simulink model "pulse_heating_official_spine_v04"  (R2025b)
settings: Solver=VariableStepAuto  StartTime=0.0  StopTime=0.25  RelTol=1e-3
PreLoadFcn:
  | addpath('C:\Users\ADMIN\Documents\MATLAB\Examples\R2025b\simscapeelectrical\BatteryThermalManagementExample');
  | addpath('C:\Users\ADMIN\Documents\MATLAB\Examples\R2025b\mcb\SIUnitsExample');
  | addpath('C:\Users\ADMIN\Documents\MATLAB\Examples\R2025b\simscapeelectrical\PMSMDriveThermalExample');
  | load_system('PMSMDriveThermal');
  | set_param('PMSMDriveThermal','SimscapeLogType','none','SimscapeLogSimulationStatistics','off');
  | set_param('PMSMDriveThermal','Dirty','off');
InitFcn:
  | % === M4-02A: Clean parameter matching (MO theory PI) ===
  | addpath('C:\Users\ADMIN\Documents\MATLAB\Examples\R2025b\simscapeelectrical\BatteryThermalManagementExample');
  | addpath('C:\Users\ADMIN\Documents\MATLAB\Examples\R2025b\mcb\SIUnitsExample');
  | addpath('C:\Users\ADMIN\Documents\MATLAB\Examples\R2025b\simscapeelectrical\PMSMDriveThermalExample');
  | load_system('PMSMDriveThermal');
  | PMSMDriveThermalData;
  | mcb_pmsm_foc_qep_f28379d_SIUnit_data;
  | clearvars('all');
  | 
  | % --- Construct clean pmsm struct from PMSMDriveThermal ---
  | pmsm = struct();
  | pmsm.Rs = Rs; pmsm.Ld = Ld; pmsm.Lq = Lq; pmsm.p = N; pmsm.FluxPM = PM;
  | pmsm.J = J; pmsm.B = 2.6369e-6; pmsm.I_rated = Imax;
  | pmsm.Ke = PM*N; pmsm.Kt = 1.5*N*PM; pmsm.N_max = 60*fnom/N;
  | pmsm.PositionOffset = 0; pmsm.QEPSlits = 1000;
  | 
  | inverter.V_dc = 70; dataType = 'double';
  | pmsm.N_base = inverter.V_dc / (sqrt(3)*PM*N*2*pi/60);
  | pmsm.T_rated = 1.5*N*PM*Imax;
  | 
  | % --- Timing (PMSMDriveThermal semantics) ---
  | Ts = 2e-6; fsw = 2e3; fc = fsw*10; Tsc = 1/fc;
  | T_pwm = 1/fsw; PWM_frequency = fsw; Ts_simulink = Tsc;
  | Ts_motor = Tsc; Ts_speed = 10*Tsc; Ts_inverter = Tsc;
  | 
  | % --- PI gains via mcb.calcFOCGains (MO theory) ---
  | motor = pmsm; motor.Rs = pmsm.Rs + inverter.R_board;
  | PI_params = mcb.calcFOCGains(motor, Tsc, Ts_speed, SpdLPFltCoeff=0.01);
  | PI_params.delay_Currents = int32(1);
  | PI_params.delay_Position = int32(1);
  | 
  | BatteryThermalManagementInitialization;
  | ambient = 263.15; coolantTemp = 263.15;
  | cellT_ini = ambient*ones(1,Ns*Np); cellT_ini4 = ambient*ones(1,Ns4*Np4);
  | Ns_total = 3*Ns + Ns4; Np_total = Np;
  | R_pack = Ns_total * R0_mat(3,2) / Np_total;
  | I_base_A = AH * Np_total; V_pack_nom = Ns_total * 3.3;
  | 
  | % === M4-01 generalized Reference / Platform contract ===
  | % Values are traceable engineering/platform defaults, not device ratings.
  | ReferenceConfig_ID = 'M4-01-REF-PLATFORM-v02';
  | ReferenceConfig_Source = 'OFFICIAL+ENGINEERING_DEFAULT';
  | ReferenceConfig_Scope = 'generalized_system_integration';
  | HVPath_R = 0.01;
  | DCLink_C = 470e-6;
  | DCLink_V0 = 0;
  | RMS_Window_s = 20/fsw;
  | IGBT_Ron_ref = 1e-3;
  | IGBT_Vf_ref = 1.2;
  | 
  | % Encoder/reference topology provides the static mechanical boundary.
  | OpenLoop_Vabc_Scale = 1;
model workspace (MAT data in the model file):
  control_status_v4d2_partial_duty_code = 6
  diagnostic_frequency_Hz = 50
  drive_status_v4d2_partial_current_code = 6
  kpi_status_v4d2_partial_numeric_code = 6
  kpi_value_unknown = nan
  limit_factor_unknown_code = 99
  limit_margin_unknown_value = nan
  limit_status_v4c_code = 5
  pulse_command_status_code = 6
  pulse_duty_percent = 50
  pulse_id_amplitude_A = 40
  pulse_iq_amplitude_A = 0
  pulse_mode_code = 4
  pulse_phase_delay_s = 0
undefined symbols (not defined in the file or in its folder): DiscIntNeverNeededParam, f_losses, Flowrate_vec, Isc_losses, losses_oc, losses_sc, N, PM, Rs
libraries: fl_lib x38, nesl_utility x35, ee_lib x12, mcbcontrolslib x5, mcbeeMathTransformLib x3, slpidlib x2, mcbhdlpositiondecoderlib x1, eePwmGeneratorTwoLevel x1
(part 1 of 4)
settings Model: Creator=ADMIN  LastModifiedBy=ADMIN
settings DataIOCC: ReturnWorkspaceOutputs=off
settings DebuggingCC: UnderspecifiedInitializationDetection=Classic
settings SimscapeCC: SimscapeLogType=all  SimscapeLogName=simlog_v4e

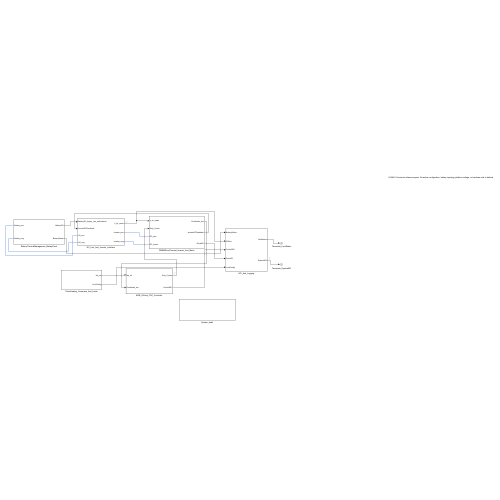
[thumbnail: Simulink's stored preview of the top-level diagram]
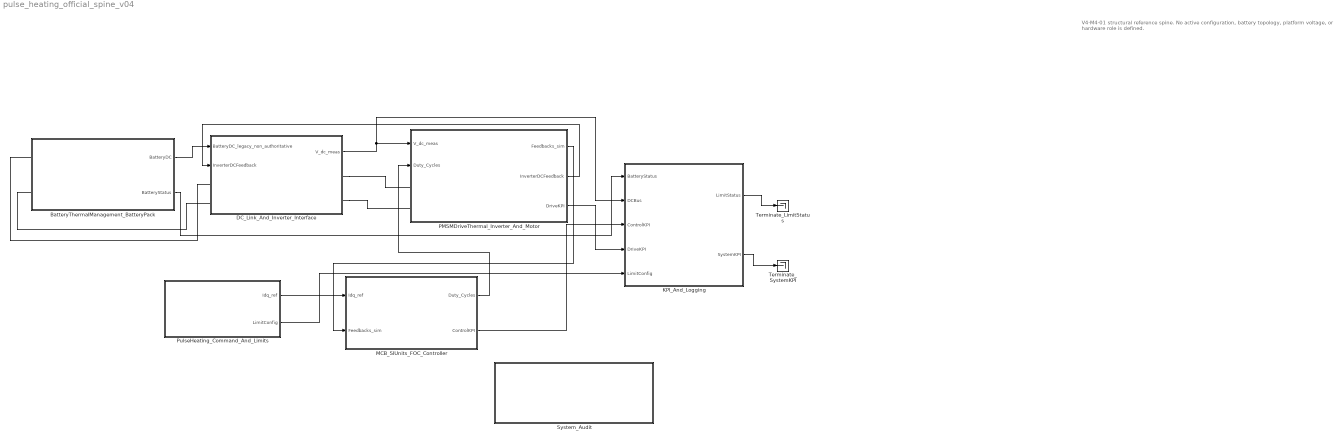
== system pulse_heating_official_spine_v04 ==
  note: V4-M4-01 structural reference spine. No active configuration, battery topology, platform voltage, or hardware role is defined.
  BatteryThermalManagement_BatteryPack : Subsystem
  DC_Link_And_Inverter_Interface : Subsystem
  KPI_And_Logging : Subsystem
  MCB_SIUnits_FOC_Controller : Subsystem
  PMSMDriveThermal_Inverter_And_Motor : Subsystem
  PulseHeating_Command_And_Limits : Subsystem
  System_Audit : Subsystem
  Terminate_LimitStatus : Terminator
  Terminate_SystemKPI : Terminator
  wires:
  BatteryThermalManagement_BatteryPack/1(BatteryDC) -> DC_Link_And_Inverter_Interface/1(BatteryDC_legacy_non_authoritative)
  BatteryThermalManagement_BatteryPack/2(BatteryStatus) -> KPI_And_Logging/1(BatteryStatus)
  PMSMDriveThermal_Inverter_And_Motor/2(InverterDCFeedback) -> DC_Link_And_Inverter_Interface/2(InverterDCFeedback)
  PMSMDriveThermal_Inverter_And_Motor/1(Feedbacks_sim) -> MCB_SIUnits_FOC_Controller/2(Feedbacks_sim)
  PMSMDriveThermal_Inverter_And_Motor/3(DriveKPI) -> KPI_And_Logging/4(DriveKPI)
  PulseHeating_Command_And_Limits/1(Idq_ref) -> MCB_SIUnits_FOC_Controller/1(Idq_ref)
  PulseHeating_Command_And_Limits/2(LimitConfig) -> KPI_And_Logging/5(LimitConfig)
  KPI_And_Logging/1(LimitStatus) -> Terminate_LimitStatus/1
  DC_Link_And_Inverter_Interface/1(V_dc_meas) -> PMSMDriveThermal_Inverter_And_Motor/1(V_dc_meas), KPI_And_Logging/2(DCBus)
  MCB_SIUnits_FOC_Controller/1(Duty_Cycles) -> PMSMDriveThermal_Inverter_And_Motor/2(Duty_Cycles)
  MCB_SIUnits_FOC_Controller/2(ControlKPI) -> KPI_And_Logging/3(ControlKPI)
  KPI_And_Logging/2(SystemKPI) -> Terminate_SystemKPI/1
  connections:
  BatteryThermalManagement_BatteryPack/LConn2 -- DC_Link_And_Inverter_Interface/LConn2
  BatteryThermalManagement_BatteryPack/LConn1 -- DC_Link_And_Inverter_Interface/LConn1
  DC_Link_And_Inverter_Interface/RConn1 -- PMSMDriveThermal_Inverter_And_Motor/LConn1
  DC_Link_And_Inverter_Interface/RConn2 -- PMSMDriveThermal_Inverter_And_Motor/LConn2

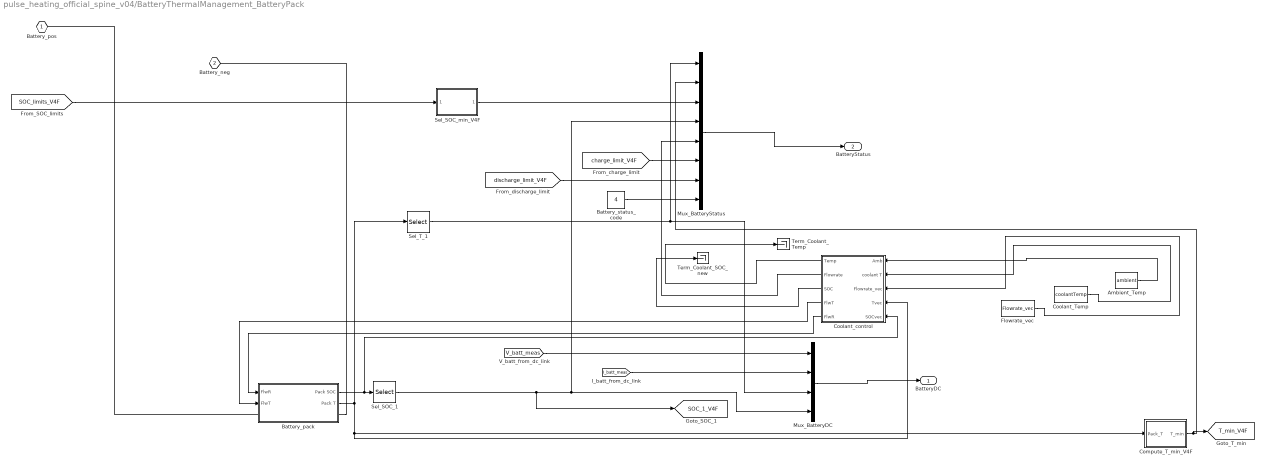
== system pulse_heating_official_spine_v04/BatteryThermalManagement_BatteryPack ==
  Ambient_Temp : Constant  Value=ambient
  Battery_pack : Subsystem
  Battery_status_code : Constant  Value=4
  Compute_T_min_V4F : MATLAB Function  TreatAsAtomicUnit=on
  Coolant_Temp : Constant  Value=coolantTemp
  Coolant_control : Subsystem
  Flowrate_vec : Constant  Value=Flowrate_vec
  Mux_BatteryDC : Mux
  Mux_BatteryStatus : Mux  Inputs=8
  Sel_SOC_1 : Selector  InputPortWidth=42  IndexOptions=Index vector (dialog)  Indices=1  OutputSizes=1
  Sel_SOC_min_V4F : MATLAB Function  TreatAsAtomicUnit=on
  Sel_T_1 : Selector  InputPortWidth=42  IndexOptions=Index vector (dialog)  Indices=1  OutputSizes=1
  Term_Coolant_SOC_new : Terminator
  Term_Coolant_Temp : Terminator
  Battery_pos : PMIOPort  Side=Left
  Battery_neg : PMIOPort  Port=2  Side=Left
  BatteryDC : Outport
  BatteryStatus : Outport  Port=2
  tag scope: SOC_1_V4F=global, T_min_V4F=global
  wires:
  Compute_T_min_V4F/1(T_min) -> [T_min_V4F], Mux_BatteryStatus/2
  Battery_pack/2(Pack T) -> Coolant_control/4(Tvec), Compute_T_min_V4F/1(Pack_T), Sel_T_1/1
  Battery_pack/1(Pack SOC) -> Coolant_control/5(SOCvec), Sel_SOC_1/1
  Flowrate_vec/1 -> Coolant_control/3(Flowrate_vec)
  Coolant_Temp/1 -> Coolant_control/2(coolant T)
  Ambient_Temp/1 -> Coolant_control/1(Amb)
  Coolant_control/1(Temp) -> Term_Coolant_Temp/1
  Coolant_control/3(SOC) -> Term_Coolant_SOC_new/1
  Coolant_control/4(FlwT) -> Battery_pack/2(FlwT)
  Mux_BatteryDC/1 -> BatteryDC/1
  Coolant_control/5(FlwR) -> Battery_pack/1(FlwR)
  Mux_BatteryStatus/1 -> BatteryStatus/1
  Sel_SOC_1/1 -> Mux_BatteryDC/4, Mux_BatteryStatus/4, [SOC_1_V4F]
  [I_batt_meas] -> Mux_BatteryDC/2
  Sel_T_1/1 -> Mux_BatteryStatus/1, Mux_BatteryDC/3
  [V_batt_meas] -> Mux_BatteryDC/1
  Battery_status_code/1 -> Mux_BatteryStatus/8
  [charge_limit_V4F] -> Mux_BatteryStatus/6
  Sel_SOC_min_V4F/1(SOC_min) -> Mux_BatteryStatus/3
  [SOC_limits_V4F] -> Sel_SOC_min_V4F/1(SOC_limits)
  Coolant_control/2(Flowrate) -> Mux_BatteryStatus/5
  [discharge_limit_V4F] -> Mux_BatteryStatus/7
  connections:
  Battery_pack/LConn1 -- Battery_pos/RConn1
  Battery_pack/RConn1 -- Battery_neg/RConn1

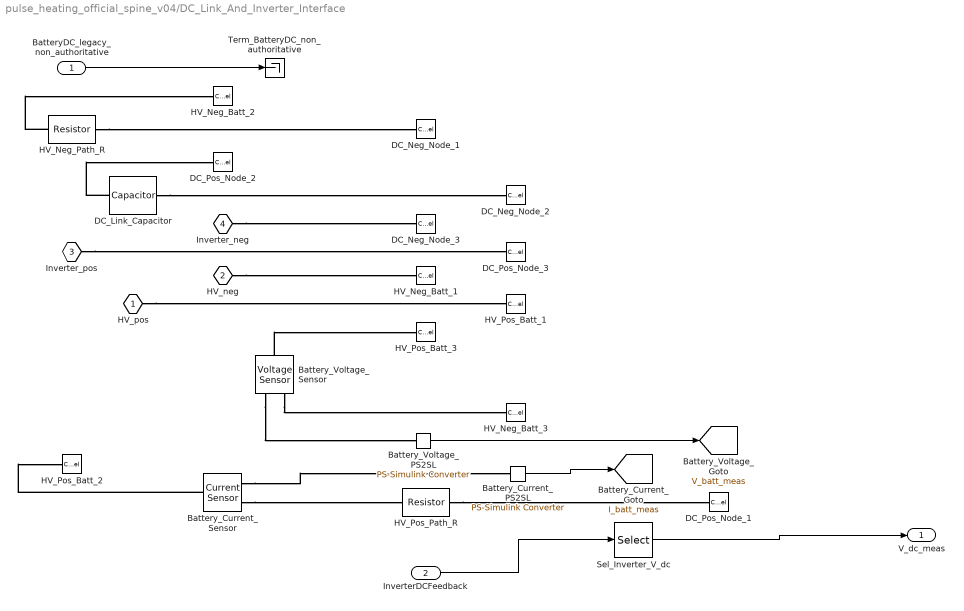
== system pulse_heating_official_spine_v04/DC_Link_And_Inverter_Interface ==
  BatteryDC_legacy_non_authoritative : Inport
  InverterDCFeedback : Inport  Port=2
  Battery_Current_PS2SL : nesl_utility/PS-Simulink Converter  PhysicalDomain=network_engine_domain  SubClassName=ps_output  LeftPortType=input  RightPortType=output  PseudoPeriodic=off  Frequencies=[]  VectorFormat=inherit  Unit=inherit  AffineConversion=off
  Battery_Current_Sensor : fl_lib/Electrical/Electrical Sensors/Current Sensor
  Battery_Voltage_PS2SL : nesl_utility/PS-Simulink Converter  PhysicalDomain=network_engine_domain  SubClassName=ps_output  LeftPortType=input  RightPortType=output  PseudoPeriodic=off  Frequencies=[]  VectorFormat=inherit  Unit=inherit  AffineConversion=off
  Battery_Voltage_Sensor : fl_lib/Electrical/Electrical Sensors/Voltage Sensor
  DC_Link_Capacitor : ee_lib/Passive/Capacitor  cap_option=ee.enum.passive.capacitor.capOption.const  c=DCLink_C F  Cvec=[1e-05, 1e-06] F  Vvec=[0, 10] V  CV_table_symmetry=ee.enum.passive.capacitor.tableSymmetry.yes  f_vec=[1, 10] kHz  DFext_vec=[.8, 1.2]  enable_C_tol=ee.enum.toleranceApplication.none  averaging_period=0 s  C_tol=5  tol_distribution=ee.enum.toleranceDistribution.uniform  nSigma=4  r=0 Ohm  g=0 1/Ohm  enable_operating_limits=ee.enum.enable.no  operating_limit_action=ee.enum.passive.reportOpLim.warn  max_working_voltage_range=[-25, 25] V  power_rating=1 W  maxTemperature=85 degC  thermalEnable=false  thermalMass=1 J/K  i_specify=off  i_priority=None  i=0 A  i_nominal_specify=off  i_nominal_value=1  i_nominal_unit=A  v_specify=off  v_priority=None  v=DCLink_V0 V  v_nominal_specify=off  v_nominal_value=1  v_nominal_unit=V  vc_specify=off  vc_priority=High  vc=DCLink_V0 V  vc_nominal_specify=off  vc_nominal_value=1  vc_nominal_unit=V  T_specify=off  T_priority=None  T=298.15 K  T_nominal_specify=off  T_nominal_value=1  T_nominal_unit=K
  DC_Neg_Node_1 : ConnectionLabel  Label=DC_NEG_NODE
  DC_Neg_Node_2 : ConnectionLabel  Label=DC_NEG_NODE
  DC_Neg_Node_3 : ConnectionLabel  Label=DC_NEG_NODE
  DC_Pos_Node_1 : ConnectionLabel  Label=DC_POS_NODE
  DC_Pos_Node_2 : ConnectionLabel  Label=DC_POS_NODE
  DC_Pos_Node_3 : ConnectionLabel  Label=DC_POS_NODE
  HV_Neg_Batt_1 : ConnectionLabel  Label=HV_NEG_BATT_NODE
  HV_Neg_Batt_2 : ConnectionLabel  Label=HV_NEG_BATT_NODE
  HV_Neg_Batt_3 : ConnectionLabel  Label=HV_NEG_BATT_NODE
  HV_Neg_Path_R : ee_lib/Passive/Resistor  R=HVPath_R Ohm  enable_R_tol=ee.enum.toleranceApplication.none  R_tol=5  tol_distribution=ee.enum.toleranceDistribution.uniform  nSigma=4  enable_operating_limits=ee.enum.enable.no  operating_limit_action=ee.enum.passive.reportOpLim.warn  power_rating=1 W  max_working_voltage=100 V  noise_mode=ee.enum.sources.noise.Disabled  Tdevice=25 degC  sample_time=1e-3 s  repeatability=ee.enum.ic.repeatability.notRepeatable  user_seed=0  auto_seed=3922919431  power_derating_T1=70 degC  power_derating_T2=155 degC  operating_temperature_range_vec=[-50, 150] degC  alpha=3.93e-3 1/K  Tmeas=25 degC  thermal_mass=100 J/K  temperature_specify=off  temperature_priority=High  temperature=298.15 K  temperature_nominal_specify=off  temperature_nominal_value=1  temperature_nominal_unit=K
  HV_Pos_Batt_1 : ConnectionLabel  Label=HV_POS_BATT_NODE
  HV_Pos_Batt_2 : ConnectionLabel  Label=HV_POS_BATT_NODE
  HV_Pos_Batt_3 : ConnectionLabel  Label=HV_POS_BATT_NODE
  HV_Pos_Path_R : ee_lib/Passive/Resistor  R=HVPath_R Ohm  enable_R_tol=ee.enum.toleranceApplication.none  R_tol=5  tol_distribution=ee.enum.toleranceDistribution.uniform  nSigma=4  enable_operating_limits=ee.enum.enable.no  operating_limit_action=ee.enum.passive.reportOpLim.warn  power_rating=1 W  max_working_voltage=100 V  noise_mode=ee.enum.sources.noise.Disabled  Tdevice=25 degC  sample_time=1e-3 s  repeatability=ee.enum.ic.repeatability.notRepeatable  user_seed=0  auto_seed=545404223  power_derating_T1=70 degC  power_derating_T2=155 degC  operating_temperature_range_vec=[-50, 150] degC  alpha=3.93e-3 1/K  Tmeas=25 degC  thermal_mass=100 J/K  temperature_specify=off  temperature_priority=High  temperature=298.15 K  temperature_nominal_specify=off  temperature_nominal_value=1  temperature_nominal_unit=K
  Sel_Inverter_V_dc : Selector  InputPortWidth=4  IndexOptions=Index vector (dialog)  Indices=1  OutputSizes=1
  Term_BatteryDC_non_authoritative : Terminator
  HV_pos : PMIOPort  Side=Left
  HV_neg : PMIOPort  Port=2  Side=Left
  Inverter_pos : PMIOPort  Port=3  Side=Right
  Inverter_neg : PMIOPort  Port=4  Side=Right
  V_dc_meas : Outport
  tag scope: I_batt_meas=global, V_batt_meas=global
  wires:
  BatteryDC_legacy_non_authoritative/1 -> Term_BatteryDC_non_authoritative/1
  InverterDCFeedback/1 -> Sel_Inverter_V_dc/1
  Sel_Inverter_V_dc/1 -> V_dc_meas/1
  Battery_Current_PS2SL/1 -> [I_batt_meas]
  Battery_Voltage_PS2SL/1 -> [V_batt_meas]
  connections:
  Battery_Current_Sensor/RConn2 -- HV_Pos_Path_R/LConn1
  Battery_Current_Sensor/RConn1 -- Battery_Current_PS2SL/LConn1
  Battery_Voltage_Sensor/RConn1 -- Battery_Voltage_PS2SL/LConn1
  HV_pos/RConn1 -- HV_Pos_Batt_1/LConn1
  Battery_Current_Sensor/LConn1 -- HV_Pos_Batt_2/LConn1
  Battery_Voltage_Sensor/LConn1 -- HV_Pos_Batt_3/LConn1
  HV_neg/RConn1 -- HV_Neg_Batt_1/LConn1
  HV_Neg_Path_R/LConn1 -- HV_Neg_Batt_2/LConn1
  Battery_Voltage_Sensor/RConn2 -- HV_Neg_Batt_3/LConn1
  HV_Pos_Path_R/RConn1 -- DC_Pos_Node_1/LConn1
  DC_Link_Capacitor/LConn1 -- DC_Pos_Node_2/LConn1
  Inverter_pos/RConn1 -- DC_Pos_Node_3/LConn1
  HV_Neg_Path_R/RConn1 -- DC_Neg_Node_1/LConn1
  DC_Link_Capacitor/RConn1 -- DC_Neg_Node_2/LConn1
  Inverter_neg/RConn1 -- DC_Neg_Node_3/LConn1

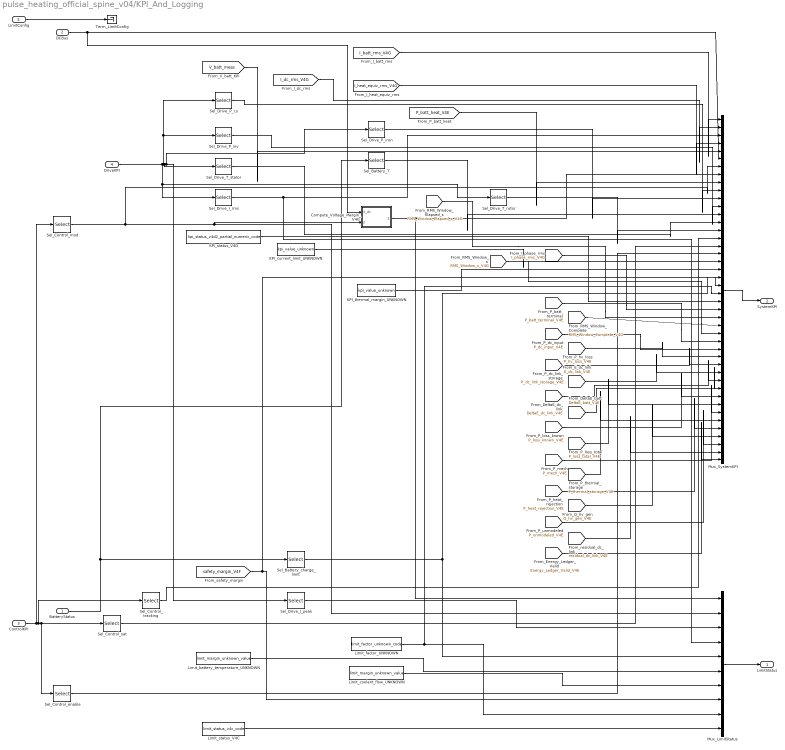
== system pulse_heating_official_spine_v04/KPI_And_Logging ==
  BatteryStatus : Inport
  DCBus : Inport  Port=2
  ControlKPI : Inport  Port=3
  DriveKPI : Inport  Port=4
  LimitConfig : Inport  Port=5
  Compute_Voltage_Margin_V4G : MATLAB Function  TreatAsAtomicUnit=on
  KPI_current_limit_UNKNOWN : Constant  Value=kpi_value_unknown
  KPI_status_V4D : Constant  Value=kpi_status_v4d2_partial_numeric_code
  KPI_thermal_margin_UNKNOWN : Constant  Value=kpi_value_unknown
  Limit_battery_temperature_UNKNOWN : Constant  Value=limit_margin_unknown_value
  Limit_coolant_flow_UNKNOWN : Constant  Value=limit_margin_unknown_value
  Limit_factor_UNKNOWN : Constant  Value=limit_factor_unknown_code
  Limit_status_V4C : Constant  Value=limit_status_v4c_code
  Mux_LimitStatus : Mux  Inputs=10
  Mux_SystemKPI : Mux  Inputs=44
  Sel_Battery_T : Selector  InputPortWidth=8  IndexOptions=Index vector (dialog)  Indices=1  OutputSizes=1
  Sel_Battery_charge_limit : Selector  InputPortWidth=8  IndexOptions=Index vector (dialog)  Indices=6  OutputSizes=1
  Sel_Control_enable : Selector  InputPortWidth=5  IndexOptions=Index vector (dialog)  Indices=4  OutputSizes=1
  Sel_Control_mod : Selector  InputPortWidth=5  IndexOptions=Index vector (dialog)  Indices=2  OutputSizes=1
  Sel_Control_sat : Selector  InputPortWidth=5  IndexOptions=Index vector (dialog)  Indices=3  OutputSizes=1
  Sel_Control_tracking : Selector  InputPortWidth=5  IndexOptions=Index vector (dialog)  Indices=1  OutputSizes=1
  Sel_Drive_I_peak : Selector  InputPortWidth=8  IndexOptions=Index vector (dialog)  Indices=2  OutputSizes=1
  Sel_Drive_I_rms : Selector  InputPortWidth=8  IndexOptions=Index vector (dialog)  Indices=1  OutputSizes=1
  Sel_Drive_P_cu : Selector  InputPortWidth=8  IndexOptions=Index vector (dialog)  Indices=3  OutputSizes=1
  Sel_Drive_P_inv : Selector  InputPortWidth=8  IndexOptions=Index vector (dialog)  Indices=5  OutputSizes=1
  Sel_Drive_P_iron : Selector  InputPortWidth=8  IndexOptions=Index vector (dialog)  Indices=4  OutputSizes=1
  Sel_Drive_T_rotor : Selector  InputPortWidth=8  IndexOptions=Index vector (dialog)  Indices=7  OutputSizes=1
  Sel_Drive_T_stator : Selector  InputPortWidth=8  IndexOptions=Index vector (dialog)  Indices=6  OutputSizes=1
  Term_LimitConfig : Terminator
  LimitStatus : Outport
  SystemKPI : Outport  Port=2
  wires:
  Sel_Drive_P_cu/1 -> Mux_SystemKPI/10
  BatteryStatus/1 -> Sel_Battery_T/1, Sel_Battery_charge_limit/1
  LimitConfig/1 -> Term_LimitConfig/1
  Sel_Control_sat/1 -> Mux_SystemKPI/17
  ControlKPI/1 -> Sel_Control_enable/1, Sel_Control_sat/1, Sel_Control_tracking/1, Sel_Control_mod/1
  DCBus/1 -> Mux_SystemKPI/6, Compute_Voltage_Margin_V4G/1(V_dc)
  DriveKPI/1 -> Sel_Drive_T_rotor/1, Sel_Drive_I_rms/1, Sel_Drive_I_peak/1, Sel_Drive_P_iron/1, Sel_Drive_T_stator/1, Sel_Drive_P_inv/1, Sel_Drive_P_cu/1
  Sel_Control_mod/1 -> Compute_Voltage_Margin_V4G/2(mod_index), Mux_LimitStatus/2, Mux_SystemKPI/7
  Limit_status_V4C/1 -> Mux_LimitStatus/10
  Sel_Control_tracking/1 -> Mux_SystemKPI/16
  Sel_Control_enable/1 -> Mux_SystemKPI/18
  [I_batt_rms_V4G] -> Mux_SystemKPI/1
  [I_dc_rms_V4G] -> Mux_SystemKPI/2
  [I_heat_equiv_rms_V4G] -> Mux_SystemKPI/4
  [V_batt_meas] -> Mux_SystemKPI/5
  Mux_SystemKPI/1 -> SystemKPI/1
  [P_batt_heat_V4E] -> Mux_SystemKPI/9
  Sel_Drive_P_iron/1 -> Mux_SystemKPI/11
  Sel_Drive_P_inv/1 -> Mux_SystemKPI/12
  Sel_Battery_T/1 -> Mux_SystemKPI/13
  Sel_Drive_T_stator/1 -> Mux_SystemKPI/14
  Sel_Drive_T_rotor/1 -> Mux_SystemKPI/15
  KPI_status_V4D/1 -> Mux_SystemKPI/24
  Sel_Drive_I_rms/1 -> Mux_SystemKPI/3, Mux_LimitStatus/4
  Compute_Voltage_Margin_V4G/1(V_margin) -> Mux_LimitStatus/1, Mux_SystemKPI/8
  KPI_current_limit_UNKNOWN/1 -> Mux_SystemKPI/19
  KPI_thermal_margin_UNKNOWN/1 -> Mux_SystemKPI/20
  Limit_coolant_flow_UNKNOWN/1 -> Mux_LimitStatus/7
  Sel_Battery_charge_limit/1 -> Mux_LimitStatus/5, Mux_SystemKPI/21
  Mux_LimitStatus/1 -> LimitStatus/1
  [safety_margin_V4F] -> Mux_LimitStatus/8, Mux_SystemKPI/22
  Sel_Drive_I_peak/1 -> Mux_LimitStatus/3
  Limit_factor_UNKNOWN/1 -> Mux_SystemKPI/23, Mux_LimitStatus/9
  Limit_battery_temperature_UNKNOWN/1 -> Mux_LimitStatus/6
  [I_phase_rms_V4G] -> Mux_SystemKPI/25
  [RMS_Window_Elapsed_s_V4G] -> Mux_SystemKPI/26
  [RMS_Window_Complete_V4G] -> Mux_SystemKPI/27
  [RMS_Window_s_V4G] -> Mux_SystemKPI/28
  [P_batt_terminal_V4E] -> Mux_SystemKPI/29
  [P_dc_input_V4E] -> Mux_SystemKPI/30
  [P_hv_loss_V4E] -> Mux_SystemKPI/31
  [P_dc_link_storage_V4E] -> Mux_SystemKPI/32
  [E_dc_link_V4E] -> Mux_SystemKPI/33
  [DeltaE_dc_link_V4E] -> Mux_SystemKPI/34
  [DeltaE_batt_V4E] -> Mux_SystemKPI/35
  [P_loss_known_V4E] -> Mux_SystemKPI/36
  [P_loss_total_V4E] -> Mux_SystemKPI/37
  [P_mech_V4E] -> Mux_SystemKPI/38
  [P_thermal_storage_V4E] -> Mux_SystemKPI/39
  [P_heat_rejection_V4E] -> Mux_SystemKPI/40
  [Q_hv_gen_V4E] -> Mux_SystemKPI/41
  [P_unmodeled_V4E] -> Mux_SystemKPI/42
  [residual_dc_link_V4E] -> Mux_SystemKPI/43
  [Energy_Ledger_Valid_V4E] -> Mux_SystemKPI/44

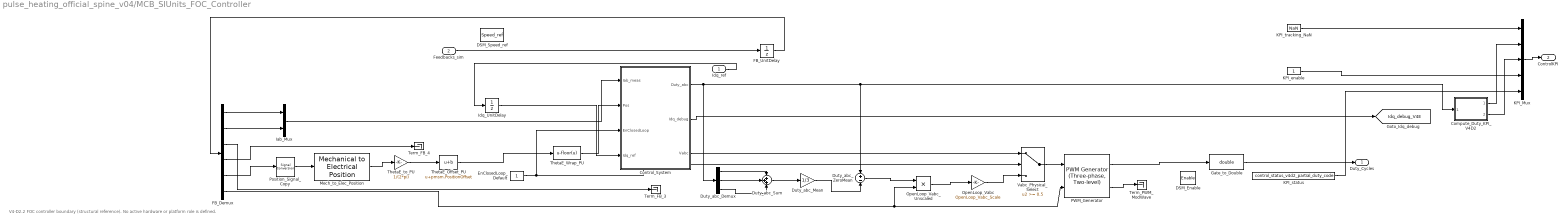
== system pulse_heating_official_spine_v04/MCB_SIUnits_FOC_Controller ==
  note: V4-D2.2 FOC controller boundary (structural reference). No active hardware or platform role is defined.
  Idq_ref : Inport
  Feedbacks_sim : Inport  Port=2
  Compute_Duty_KPI_V4D2 : MATLAB Function  TreatAsAtomicUnit=on
  Control_System : Subsystem  TreatAsAtomicUnit=on
  DSM_Enable : DataStoreMemory  DataStoreName=Enable  WriteAfterWriteMsg=warning  InitialValue=1  ShowAdditionalParam=off
  DSM_Speed_ref : DataStoreMemory  DataStoreName=Speed_ref  WriteAfterWriteMsg=warning  ShowAdditionalParam=off
  Duty_abc_Demux : Demux  Outputs=3
  Duty_abc_Mean : Gain  Gain=1/3
  Duty_abc_Sum : Sum  Inputs=+++
  Duty_abc_ZeroMean : Sum  Inputs=+-
  EnClosedLoop_Default : Constant
  FB_Demux : Demux  Outputs=6
  FB_UnitDelay : UnitDelay  InitialCondition=[0;0;0;0;0;inverter.V_dc]  SampleTime=Tsc  HasFrameUpgradeWarning=on
  Gate_to_Double : DataTypeConversion  OutDataTypeStr=double
  Iab_Mux : Mux  Inputs=2
  Idq_UnitDelay : UnitDelay  SampleTime=Tsc  HasFrameUpgradeWarning=on
  KPI_Mux : Mux  Inputs=5
  KPI_enable : Constant
  KPI_status : Constant  Value=control_status_v4d2_partial_duty_code
  KPI_tracking_NaN : Constant  Value=NaN
  Mech_to_Elec_Position : mcbhdlpositiondecoderlib/Mechanical to Electrical Position  PolePairsInputType=Specify via dialog  NrPP=pmsm.p  selectedRange=Radians  MechOfstInputType=Specify via dialog  mechOffsetIn=0  maxAngleIn=2*pi  InputDataType=double  VariantSelect=floating-point
      settings: LibrarySourceBlock=mcbhdllib/Sensor Decoders/Mechanical to Electrical Position
  OpenLoop_Vabc : Gain  Gain=OpenLoop_Vabc_Scale
  OpenLoop_Vabc_Unscaled : Product  Inputs=**
  PWM_Generator : eePwmGeneratorTwoLevel/PWM Generator (Three-phase, Two-level)  PWMMode=Continuous PWM (CPWM)  CPWMMode=SVM: space vector modulation  DPWMMode=60 DPWM: 60 degree discontinuous PWM  fsw=fsw  Ts=Ts
  Position_Signal_Copy : SignalConversion  OverrideOpt=off
  Term_FB_3 : Terminator
  Term_FB_4 : Terminator
  Term_PWM_ModWave : Terminator
  ThetaE_Offset_PU : Bias  Bias=pmsm.PositionOffset
  ThetaE_Wrap_PU : Fcn  Expr=u-floor(u)
  ThetaE_to_PU : Gain  Gain=1/(2*pi)
  Vabc_Physical_Select : Switch  Threshold=0.5
  Duty_Cycles : Outport
  ControlKPI : Outport  Port=2
  tag scope: Idq_debug_V4E=global
  wires:
  Position_Signal_Copy/1 -> Mech_to_Elec_Position/1
  FB_Demux/5 -> Position_Signal_Copy/1
  Gate_to_Double/1 -> Duty_Cycles/1
  PWM_Generator/1 -> Gate_to_Double/1
  PWM_Generator/2 -> Term_PWM_ModWave/1
  Control_System/3(Vabc) -> Vabc_Physical_Select/1
  KPI_status/1 -> KPI_Mux/5
  KPI_enable/1 -> KPI_Mux/4
  Compute_Duty_KPI_V4D2/2(sat_flag) -> KPI_Mux/3
  Compute_Duty_KPI_V4D2/1(mod_index) -> KPI_Mux/2
  KPI_Mux/1 -> ControlKPI/1
  Control_System/2(Idq_debug) -> [Idq_debug_V4E]
  Idq_UnitDelay/1 -> Control_System/4(Idq_ref)
  EnClosedLoop_Default/1 -> Control_System/3(EnClosedLoop), Vabc_Physical_Select/2
  Iab_Mux/1 -> Control_System/1(Iab_meas)
  Idq_ref/1 -> Idq_UnitDelay/1
  KPI_tracking_NaN/1 -> KPI_Mux/1
  FB_Demux/6 -> PWM_Generator/2, OpenLoop_Vabc_Unscaled/2
  FB_Demux/4 -> Term_FB_4/1
  Control_System/1(Duty_abc) -> Compute_Duty_KPI_V4D2/1(duty_abc), Duty_abc_ZeroMean/1, Duty_abc_Demux/1
  FB_Demux/3 -> Term_FB_3/1
  FB_Demux/2 -> Iab_Mux/2
  FB_UnitDelay/1 -> FB_Demux/1
  FB_Demux/1 -> Iab_Mux/1
  Feedbacks_sim/1 -> FB_UnitDelay/1
  Mech_to_Elec_Position/1 -> ThetaE_to_PU/1
  ThetaE_to_PU/1 -> ThetaE_Offset_PU/1
  ThetaE_Offset_PU/1 -> ThetaE_Wrap_PU/1
  ThetaE_Wrap_PU/1 -> Control_System/2(Pos)
  Duty_abc_Demux/1 -> Duty_abc_Sum/1
  Duty_abc_Demux/2 -> Duty_abc_Sum/2
  Duty_abc_Demux/3 -> Duty_abc_Sum/3
  Duty_abc_Sum/1 -> Duty_abc_Mean/1
  Duty_abc_Mean/1 -> Duty_abc_ZeroMean/2
  Duty_abc_ZeroMean/1 -> OpenLoop_Vabc_Unscaled/1
  OpenLoop_Vabc_Unscaled/1 -> OpenLoop_Vabc/1
  OpenLoop_Vabc/1 -> Vabc_Physical_Select/3
  Vabc_Physical_Select/1 -> PWM_Generator/1

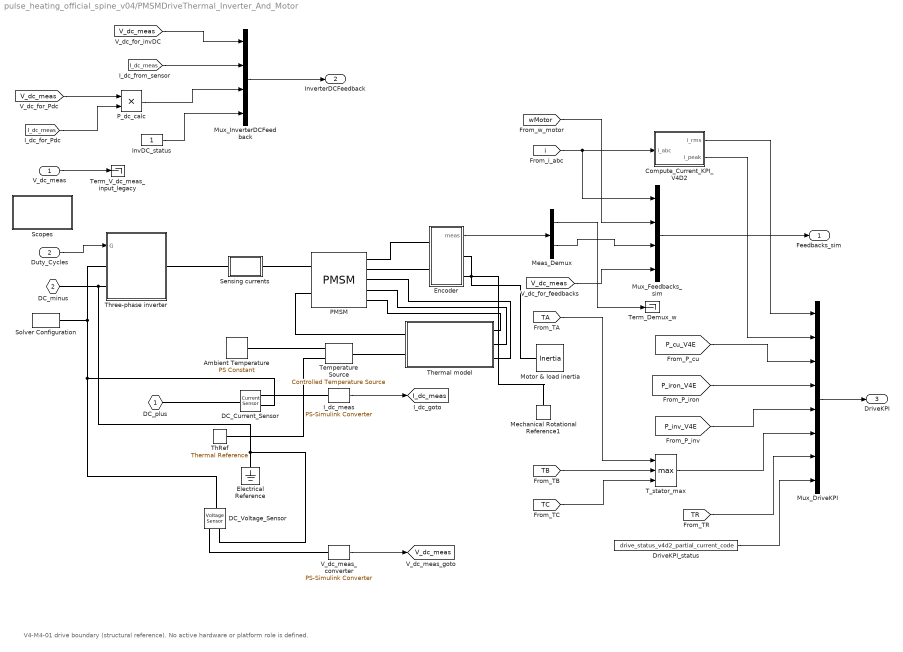
== system pulse_heating_official_spine_v04/PMSMDriveThermal_Inverter_And_Motor ==
  note: V4-M4-01 drive boundary (structural reference). No active hardware or platform role is defined.
  V_dc_meas : Inport
  Duty_Cycles : Inport  Port=2
  Ambient Temperature : fl_lib/Physical Signals/Sources/PS Constant  constant=300.15 K
  Compute_Current_KPI_V4D2 : MATLAB Function  TreatAsAtomicUnit=on
  DC_Current_Sensor : fl_lib/Electrical/Electrical Sensors/Current Sensor
  DC_Voltage_Sensor : fl_lib/Electrical/Electrical Sensors/Voltage Sensor
  DriveKPI_status : Constant  Value=drive_status_v4d2_partial_current_code
  Electrical Reference : fl_lib/Electrical/Electrical Elements/Electrical Reference
  Encoder : Subsystem
  I_dc_meas : nesl_utility/PS-Simulink Converter  PhysicalDomain=network_engine_domain  SubClassName=ps_output  LeftPortType=input  RightPortType=output  PseudoPeriodic=off  Frequencies=[]  VectorFormat=inherit  Unit=inherit  AffineConversion=off
  InvDC_status : Constant
  Meas_Demux : Demux  Outputs=2
  Mechanical Rotational Reference1 : fl_lib/Mechanical/Rotational Elements/Mechanical Rotational Reference
  Motor & load inertia : fl_lib/Mechanical/Rotational Elements/Inertia  inertia=J kg*m^2  num_ports=foundation.enum.numPorts2.one  w_specify=on  w_priority=High  w=0 rpm  w_nominal_specify=off  w_nominal_value=1  w_nominal_unit=rad/s  t_specify=off  t_priority=High  t=0 N*m  t_nominal_specify=off  t_nominal_value=1  t_nominal_unit=N*m
  Mux_DriveKPI : Mux  Inputs=8
  Mux_Feedbacks_sim : Mux
  Mux_InverterDCFeedback : Mux
  PMSM : ee_lib/Electromechanical/Permanent Magnet/PMSM  port_option=ee.enum.threePhasePort.composite  winding_type=ee.enum.statorconnection.wye  machine_param=ee.enum.pmsm.parameterization.constant  nPolePairs=N  pmflux_param=ee.enum.pmflux.fluxlinkage  pm_flux_linkage=PM Wb  torque_constant=0.18 N*m/A  back_emf_constant=0.18 V/(rad/s)  stator_param=ee.enum.statorparam.LdLqL0  Ld=Ld H  Lq=Lq H  idVec=[-200, 0, 200] A  iqVec=[-200, 0, 200] A  LdMatrix=0.0002 * ones(3, 3) H  LqMatrix=0.0002 * ones(3, 3) H  PmMatrix=0.1 * ones(3, 3) Wb  ktMatrix=0.18 * ones(3, 3) N*m/A  keMatrix=0.18 * ones(3, 3) V/(rad/s)  L0=L0 H  Ls=0.0002 H  Lm=0.00002 H  Ms=0.00002 H  Rs=Rs Ohm  zero_sequence=ee.enum.park.zerosequence.exclude  axes_param=ee.enum.rotorangle.qaxis  loss_param=ee.enum.ironloss.empirical  losses_oc=losses_oc W  losses_sc=losses_sc W  f_losses=f_losses Hz  Isc_losses=Isc_losses A  J=0 kg*m^2  lam=0 N*m/(rad/s)  i_d_specify=off  i_d_priority=None  i_d=0 A  i_d_nominal_specify=off  i_d_nominal_value=1  i_d_nominal_unit=A  i_q_specify=off  i_q_priority=None  i_q=0 A  i_q_nominal_specify=off  i_q_nominal_value=1  i_q_nominal_unit=A  torque_specify=off  torque_priority=None  torque=0 N*m  torque_nominal_specify=off  torque_nominal_value=1  torque_nominal_unit=N*m  angular_velocity_specify=on  angular_velocity_priority=None  angular_velocity=0 rpm  angular_velocity_nominal_specify=off  angular_velocity_nominal_value=1  angular_velocity_nominal_unit=rpm  angular_position_specify=on  angular_position_priority=High  angular_position=0 rad  angular_position_nominal_specify=off  angular_position_nominal_value=1  angular_position_nominal_unit=deg  alpha=alpha 1/K  alpha_flux=alpha_flux 1/K  Tmeas=Tmeas K  stator_thermal_mass=stator_thermal_mass J/K  rotor_thermal_mass=rotor_thermal_mass J/K  Rm_percent_rotor=Rm_percent_rotor  Rd_percent_rotor=Rd_percent_rotor  temperatureA_specify=off  temperatureA_priority=High  temperatureA=25 degC  temperatureA_nominal_specify=off  temperatureA_nominal_value=1  temperatureA_nominal_unit=degC  temperatureB_specify=off  temperatureB_priority=High  temperatureB=25 degC  temperatureB_nominal_specify=off  temperatureB_nominal_value=1  temperatureB_nominal_unit=degC  temperatureC_specify=off  temperatureC_priority=High  temperatureC=25 degC  temperatureC_nominal_specify=off  temperatureC_nominal_value=1  temperatureC_nominal_unit=degC  temperatureR_specify=off  temperatureR_priority=High  temperatureR=25 degC  temperatureR_nominal_specify=off  temperatureR_nominal_value=1  temperatureR_nominal_unit=degC
      settings: InternalSimscapePortConfiguration="{\"Bottom\":[],\"Left\":[{\"id\":\"N\",\"label\":\"~\",\"type\":\"foundation.electrical.three_phase\"},{\"id\":\"HR\",\"label\":\"HR\",\"type\":\"foundation.thermal.thermal\"}],\"Right\":[{\"id\":\"R\",\"label\":\"R\",\"type\":\"foundation.mechanical.rotational.rotational\"},{\"id\":\"C\",\"label\":\"C\",\"type\":\"foundation.mechanical.rotational.rotational\"},{\"id\":\"HA\",\"label\":\"HA\",\"type\":\"foundation.thermal.thermal\"},{\"id\":\"HB\",\"label\":\"HB\",\"type\":\"foundation.thermal.thermal\"},{\"id\":\"HC\",\"label\":\"HC\",\"type\":\"foundation.thermal.thermal\"}],\"Top\":[]}"
  P_dc_calc : Product
  Scopes : Subsystem
  Sensing currents : Subsystem
      mask Display: disp('i')
  Solver Configuration : nesl_utility/Solver Configuration  PhysicalDomain=network_engine_domain  SubClassName=solver  LeftPortType=input  RightPortType=generic  Tones=[]  Harmonics=[]  SimulateNoise=off  Profile=off  UseLocalSampling=off  EnableSwitchedLinearOptims=on  FrequencyDomain=off  UseCCode=off  RelTol=0.001  AbsTol=1e-06  MinStep=1e-09  ToWorkspace=off  RevertToSquareIcSolve=off  NumHomotopyIterations=100  PhasorMode=off  PhasorModeNumHarmonics=1  ConsistencySolver=NEWTON_FTOL  IndexReductionMethod=DerivativeReplacement  DoDC=off  ResidualTolerance=1e-9  ConsistencyTolSource=GLOBAL  ConsistencyAbsTol=0.001  ConsistencyRelTol=0.001  ConsistencyTolFactor=0.001  UseLocalSolver=on  LocalSolverChoice=NE_BACKWARD_EULER_ADVANCER  ResolveIndetEquations=on  FunctionEvalNumThread=1  LocalSolverSampleTime=Ts  DoFixedCost=on  MaxNonlinIter=6  MaxModeIter=2  ComputeImpulses=off  ImpulseIterations=2  LinearAlgebra=auto  LinearAlgebraNumThread=0  EquationFormulation=NE_TIME_EF  DelaysMemoryBudget=1024  AutomaticFiltering=on  FilteringTimeConstant=0.001  PartitionStorageMethod=AS_NEEDED  PartitionMemoryBudget=1024  PartitionMethod=FAST  MultibodyUseLocalSolver=off  MultibodyLocalSolverChoice=ODE1  MultibodyLocalSolverSampleTime=0.001
  T_stator_max : MinMax  Function=max  Inputs=3
  Temperature Source : fl_lib/Thermal/Thermal Sources/Controlled Temperature Source
  Term_Demux_w : Terminator
  Term_V_dc_meas_input_legacy : Terminator
  ThRef : fl_lib/Thermal/Thermal Elements/Thermal Reference
  Thermal model : Subsystem  Tag=PublishSubsystem
  Three-phase inverter : Subsystem
  V_dc_meas_converter : nesl_utility/PS-Simulink Converter  PhysicalDomain=network_engine_domain  SubClassName=ps_output  LeftPortType=input  RightPortType=output  PseudoPeriodic=off  Frequencies=[]  VectorFormat=inherit  Unit=inherit  AffineConversion=off
  DC_plus : PMIOPort  Side=Left
  DC_minus : PMIOPort  Port=2  Side=Left
  Feedbacks_sim : Outport
  InverterDCFeedback : Outport  Port=2
  DriveKPI : Outport  Port=3
  tag scope: I_dc_meas=global, V_dc_meas=global
  wires:
  [V_dc_meas] -> Mux_InverterDCFeedback/1
  [V_dc_meas] -> P_dc_calc/1
  [I_dc_meas] -> P_dc_calc/2
  [I_dc_meas] -> Mux_InverterDCFeedback/2
  V_dc_meas/1 -> Term_V_dc_meas_input_legacy/1
  Duty_Cycles/1 -> Three-phase inverter/1(G)
  P_dc_calc/1 -> Mux_InverterDCFeedback/3
  InvDC_status/1 -> Mux_InverterDCFeedback/4
  V_dc_meas_converter/1 -> [V_dc_meas]
  [P_iron_V4E] -> Mux_DriveKPI/4
  T_stator_max/1 -> Mux_DriveKPI/6
  Mux_InverterDCFeedback/1 -> InverterDCFeedback/1
  DriveKPI_status/1 -> Mux_DriveKPI/8
  Meas_Demux/2 -> Mux_Feedbacks_sim/3
  Meas_Demux/1 -> Term_Demux_w/1
  [TA] -> T_stator_max/1
  [TB] -> T_stator_max/2
  I_dc_meas/1 -> [I_dc_meas]
  Encoder/1(meas) -> Meas_Demux/1
  [wMotor] -> Mux_Feedbacks_sim/2
  [i] -> Mux_Feedbacks_sim/1, Compute_Current_KPI_V4D2/1(i_abc)
  [V_dc_meas] -> Mux_Feedbacks_sim/4
  [TC] -> T_stator_max/3
  Compute_Current_KPI_V4D2/1(i_rms) -> Mux_DriveKPI/1
  Compute_Current_KPI_V4D2/2(i_peak) -> Mux_DriveKPI/2
  Mux_Feedbacks_sim/1 -> Feedbacks_sim/1
  [P_cu_V4E] -> Mux_DriveKPI/3
  [P_inv_V4E] -> Mux_DriveKPI/5
  [TR] -> Mux_DriveKPI/7
  Mux_DriveKPI/1 -> DriveKPI/1
  connections:
  PMSM/RConn1 -- Encoder/LConn1
  PMSM/LConn2 -- Thermal model/LConn1
  Three-phase inverter/LConn1 -- DC_Current_Sensor/RConn2 -- DC_Voltage_Sensor/LConn1 -- Solver Configuration/RConn1
  DC_Voltage_Sensor/RConn2 -- Electrical Reference/LConn1 -- Three-phase inverter/LConn2 -- DC_minus/RConn1
  PMSM/RConn4 -- Thermal model/RConn2
  Three-phase inverter/RConn1 -- Sensing currents/LConn1
  DC_plus/RConn1 -- DC_Current_Sensor/LConn1
  DC_Voltage_Sensor/RConn1 -- V_dc_meas_converter/LConn1
  Sensing currents/RConn1 -- PMSM/LConn1
  Ambient Temperature/RConn1 -- Temperature Source/RConn1
  DC_Current_Sensor/RConn1 -- I_dc_meas/LConn1
  ThRef/LConn1 -- Temperature Source/RConn2
  PMSM/RConn2 -- Encoder/LConn2
  PMSM/RConn3 -- Thermal model/RConn3
  PMSM/RConn5 -- Thermal model/RConn1
  Temperature Source/LConn1 -- Thermal model/LConn2
  Encoder/RConn2 -- Encoder/RConn1 -- Motor & load inertia/LConn1 -- Mechanical Rotational Reference1/LConn1

== system pulse_heating_official_spine_v04/PulseHeating_Command_And_Limits ==
  Id_Pulse_Stall : DiscretePulseGenerator  PulseType=Time based  Period=1/diagnostic_frequency_Hz  PulseWidth=pulse_duty_percent  PhaseDelay=pulse_phase_delay_s
  Iq_ref_zero_A : Constant  Value=pulse_iq_amplitude_A
  Limit_Duty_Percent : Constant  Value=pulse_duty_percent
  Limit_Frequency_Hz : Constant  Value=diagnostic_frequency_Hz
  Limit_Id_A : Constant  Value=pulse_id_amplitude_A
  Limit_Mode_Code : Constant  Value=pulse_mode_code
  Limit_Phase_Delay_s : Constant  Value=pulse_phase_delay_s
  Limit_Status_Code : Constant  Value=pulse_command_status_code
  Mux_Idq_ref : Mux  Inputs=2
  Mux_LimitConfig : Mux  Inputs=6
  Offset_To_Negative_A : Bias  Bias=-pulse_id_amplitude_A  SaturateOnIntegerOverflow=off
  Scale_To_Bipolar_A : Gain  Gain=2*pulse_id_amplitude_A
  Idq_ref : Outport
  LimitConfig : Outport  Port=2
  wires:
  Limit_Duty_Percent/1 -> Mux_LimitConfig/3
  Limit_Id_A/1 -> Mux_LimitConfig/1
  Iq_ref_zero_A/1 -> Mux_Idq_ref/2
  Limit_Mode_Code/1 -> Mux_LimitConfig/5
  Limit_Frequency_Hz/1 -> Mux_LimitConfig/2
  Mux_LimitConfig/1 -> LimitConfig/1
  Id_Pulse_Stall/1 -> Scale_To_Bipolar_A/1
  Limit_Phase_Delay_s/1 -> Mux_LimitConfig/4
  Limit_Status_Code/1 -> Mux_LimitConfig/6
  Scale_To_Bipolar_A/1 -> Offset_To_Negative_A/1
  Offset_To_Negative_A/1 -> Mux_Idq_ref/1
  Mux_Idq_ref/1 -> Idq_ref/1

== system pulse_heating_official_spine_v04/System_Audit ==
  Battery_Envelope_Screening : Subsystem
  Energy_And_Thermal_Audit : Subsystem
  RMS_And_Measurement_Audit : Subsystem
